simulink model "ChemicalProcessOptimization"  (R2019b)
settings: Solver=FixedStepAuto  StartTime=0  StopTime=45  FixedStep=Ts  RelTol=1e-3  EnableMultiTasking=on
PreLoadFcn:
  | Ts = 0.5;
  | load CSTRData
values from neighbouring files (symbols this model uses):
  a_vec = [0.384207621232031;0.492686723524811;0.580956543031792;0.649017079752974;0.696868333688357;0.72451030483794;0.731942993201725;0.71916639877971;0.686180521571896;0.632985361578283;0.55958091879887;0.465967193233659;0.352144184882648;0.218111893745838;0.0638703198232284]    [run_benchmark.m]
  b_vec = [0.0628087670628903;0.0875474545057933;0.110088960048547;0.130433283691153;0.148580425433609;0.164530385275917;0.178283163218075;0.189838759260085;0.199197173401946;0.206358405643658;0.211322455985221;0.214089324426636;0.214659010967901;0.213031515609018;0.209206838349985]    [run_benchmark.m]
  change_per_step_Tc_control = 2    [init_vars.m]
  conc_noise = (CrEQ(1)-CrEQ(5))*noise_magnitude    [init_vars.m]
  Cr_sim_ini = 8.57    [init_vars.m]    (also in run_benchmark.m)
  Cr_vec = [2 2.5 3 3.5 4 4.5 5 5.5 6 6.5 7 7.5 8 8.5 9]    [run_benchmark.m]
  j_scenario = 1    [init_vars.m]
  Ki_vec = [-7.98512854300473;-6.23612330817463;-4.75246287755465;-3.53414725114479;-2.58117642894504;-1.8935504109554;-1.47126919717588;-1.31433278760647;-1.42274118224718;-1.796494381098;-2.43559238415893;-3.34003519142998;-4.50982280291114;-5.94495521860242;-7.64543243850381]    [run_benchmark.m]
  Kp_vec = [-2.00046148741648;-2.3184560846763;-2.65393524901532;-3.00689898043353;-3.37734727893094;-3.76528014450754;-4.17069757716334;-4.59359957689834;-5.03398614371254;-5.49185727760593;-5.96721297857851;-6.4600532466303;-6.97037808176128;-7.49818748397146;-8.04348145326083]    [run_benchmark.m]
  Kt_vec = [3.60620000481947;3.57285570622906;3.55992955218359;3.56742154268306;3.59533167772747;3.64365995731683;3.71240638145112;3.80157095013036;3.91115366335453;4.04115452112365;4.19157352343771;4.36241067029671;4.55366596170065;4.76533939764953;4.99743097814336]    [run_benchmark.m]
  Tc_sim_ini = 297.9798    [init_vars.m]
  temp_noise = (TrEQ(1)-TrEQ(5))*noise_magnitude    [init_vars.m]
  Tr_sim_ini = 311.2612    [init_vars.m]    (also in run_benchmark.m)
undefined symbols (not defined in the file or in its folder): CrEQ, DiscIntNeverNeededParam, sigbuilder_block, TrEQ
libraries: simulink x1, bonsai_library x1
settings Model: Creator=The MathWorks, Inc.  LastModifiedBy=jomcdowe
settings DataIOCC: InitialState=[311.267; 8.5695]  LimitDataPoints=on  SaveFormat=Array  ReturnWorkspaceOutputs=off  SignalLoggingName=logsOut
settings OptimizationCC: BooleanDataType=off  DefaultParameterBehavior=Inlined  InlineInvariantSignals=on  BufferReuse=off  ExpressionDepthLimit=2147483647  InitFltsAndDblsToZero=on  LifeSpan=inf
settings DebuggingCC: SaveWithParameterizedLinksMsg=none  UnderspecifiedInitializationDetection=Classic  MergeDetectMultiDrivingBlocksExec=none  CheckExecutionContextPreStartOutputMsg=on  CheckExecutionContextRuntimeOutputMsg=on  SignalResolutionControl=TryResolveAllWithWarning  MultiTaskDSMMsg=warning  MultiTaskCondExecSysMsg=none  AllowSymbolicDim=off  StateNameClashWarn=warning  SFUnexpectedBacktrackingDiag=warning  SFNoUnconditionalDefaultTransitionDiag=warning  SFExecutionAtInitializationDiag=none  ArithmeticOperatorsInVariantConditions=warning
settings HardwareCC: ProdBitPerPointer=32  ProdBitPerSizeT=32  ProdBitPerPtrDiffT=32  ProdLargestAtomicFloat=None  ProdIntDivRoundTo=Undefined  ProdEndianess=Unspecified  ProdWordSize=32  ProdHWDeviceType=32-bit Generic  TargetUnknown=on
settings ModelReferenceCC: PropagateSignalLabelsOutOfModel=off
settings SFSimCC: SimUseLocalCustomCode=off  CustomCodeUndefinedFunction=UseInterfaceOnly
settings RTWCC: RTWUseLocalCustomCode=off
settings CodeAppCC: StateflowObjectComments=on
settings GRTTargetCC: TargetFcnLib=ansi_tfl_tmw.mat  TargetLangStandard=C89/C90 (ANSI)  CombineOutputUpdateFcns=off  GRTInterface=on
settings ConfigComp: CovMetricSettings=dw  CovSaveCumulativeToWorkspaceVar=on  CovSaveSingleToWorkspaceVar=on  CovExternalEMLEnable=off  CovSFcnEnable=off

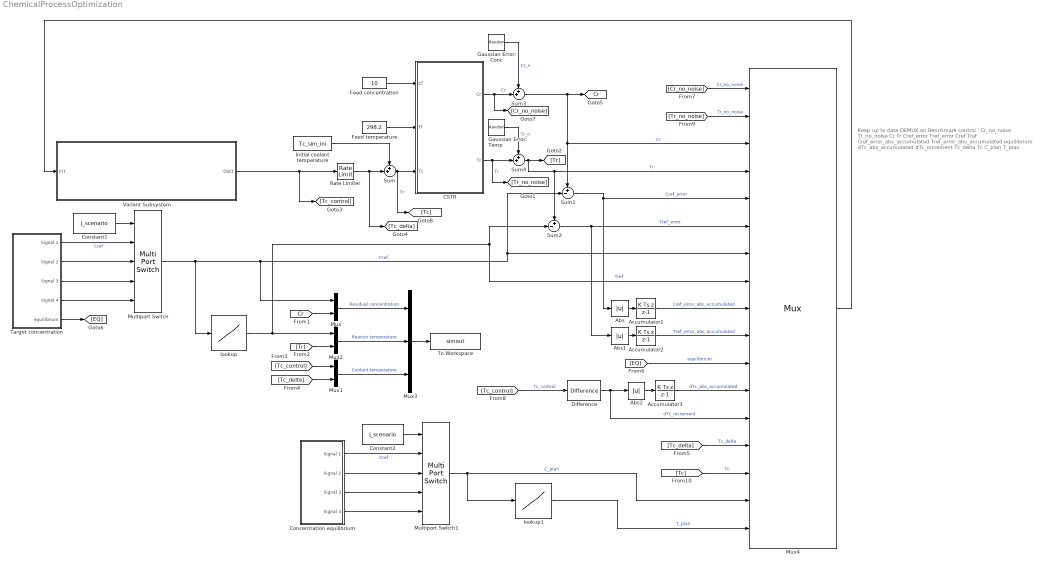
== system ChemicalProcessOptimization ==
  note: Keep up to date DEMUX on Benchmark control :
      |
      | Cr_no_noise
      | Tr_no_noise
      | Cr
      | Tr
      | Cref_error
      | Tref_error
      | Cref
      | Tref
      | Cref_error_abs_accumulated
      | Tref_error_abs_accumulated
      | equilibrium
      | dTc_abs_accumulated
      | dTc_increment
      | Tc_delta
      | Tc
      | C_plan
      | T_plan
  Abs : Abs
  Abs1 : Abs
  Abs2 : Abs
  Accumulator1 : DiscreteIntegrator  IntegratorMethod=Integration: Backward Euler  gainval=1/Ts  SampleTime=-1  ICPrevOutput=DiscIntNeverNeededParam  ICPrevScaledInput=DiscIntNeverNeededParam
  Accumulator2 : DiscreteIntegrator  IntegratorMethod=Integration: Backward Euler  gainval=1/Ts  SampleTime=-1  ICPrevOutput=DiscIntNeverNeededParam  ICPrevScaledInput=DiscIntNeverNeededParam
  Accumulator3 : DiscreteIntegrator  IntegratorMethod=Integration: Backward Euler  gainval=1/Ts  SampleTime=-1  ICPrevOutput=DiscIntNeverNeededParam  ICPrevScaledInput=DiscIntNeverNeededParam
  CSTR : Subsystem
  Concentration equilibrium : Subsystem  Tag=STV Subsys  LoadFcn=sigbuilder_block('load');  StartFcn=sigbuilder_block('start');  StopFcn=sigbuilder_block('stop');  ClipboardFcn=sigbuilder_block('clipboard');  mask(Sigbuilder block){tuvar=[0:10]}
      mask help: Simulink:masks:SigbuilderBlock_MD
      mask init:
      | if ~strcmp(get_param(bdroot(gcbh),'SimulationStatus'),'stopped') tuvar = sigbuilder_block('maskInit'); end
      settings: CopyFcn=sigbuilder_block('copy');  DeleteFcn=sigbuilder_block('delete');  ModelCloseFcn=sigbuilder_block('modelClose');  PreSaveFcn=sigbuilder_block('preSave');  PauseFcn=sigbuilder_block('pause');  ContinueFcn=sigbuilder_block('continue');  NameChangeFcn=sigbuilder_block('namechange');  OpenFcn=sigbuilder_block('open',[490.5 190.125 550.5 359.625 ]);  CloseFcn=sigbuilder_block('close');
      mask Display: plot(0, 0, 100, 100,[2, 2, 32, 32, 2], [68, 8, 8, 68, 68],[32, 2], [38, 38], [32, 19, 2],[53, 60, 44], [32, 17, 17, 2],[16, 16, 31, 31]);txt = getActiveGroup(gcbh);text(2, 100, txt,'verticalAlignment', 'top');
  Constant1 : Constant  Value=j_scenario
  Constant2 : Constant  Value=j_scenario
  Difference : simulink/Discrete/Difference  ICPrevInput=0.0  OutMin=[]  OutMax=[]  OutDataType=fixdt(1, 16)  OutScaling=2^-10  DoSatur=off
  Feed concentration : Constant  Value=10  SampleTime=0
  Feed temperature : Constant  Value=298.2  SampleTime=0
  Gaussian Error: Conc : RandomNumber  Variance=conc_noise*conc_noise  SampleTime=Ts
  Gaussian Error: Temp : RandomNumber  Variance=temp_noise*temp_noise  Seed=10  SampleTime=Ts
  Initial coolant temperature : Constant  Value=Tc_sim_ini  SampleTime=0
  Multiport Switch : MultiPortSwitch  Inputs=4
  Multiport Switch1 : MultiPortSwitch  Inputs=4
  Mux : Mux  Inputs=2
  Mux1 : Mux  Inputs=2
  Mux2 : Mux  Inputs=2
  Mux3 : Mux  Inputs=3
  Mux4 : Mux  Inputs=17
      settings: DisplayOption=signals
  Rate Limiter : RateLimiter  RisingSlewLimit=10  FallingSlewLimit=-10  SampleTimeMode=inherited
  Sum : Sum  Inputs=++|
  Sum1 : Sum  Inputs=+-|
  Sum2 : Sum  Inputs=+-|
  Sum3 : Sum  Inputs=++|
  Sum4 : Sum  Inputs=++|
  Target concentration : Subsystem  Tag=STV Subsys  LoadFcn=sigbuilder_block('load');  StartFcn=sigbuilder_block('start');  StopFcn=sigbuilder_block('stop');  ClipboardFcn=sigbuilder_block('clipboard');  mask(Sigbuilder block){tuvar=[0:10]}
      mask help: Simulink:masks:SigbuilderBlock_MD
      mask init:
      | if ~strcmp(get_param(bdroot(gcbh),'SimulationStatus'),'stopped') tuvar = sigbuilder_block('maskInit'); end
      settings: CopyFcn=sigbuilder_block('copy');  DeleteFcn=sigbuilder_block('delete');  ModelCloseFcn=sigbuilder_block('modelClose');  PreSaveFcn=sigbuilder_block('preSave');  PauseFcn=sigbuilder_block('pause');  ContinueFcn=sigbuilder_block('continue');  NameChangeFcn=sigbuilder_block('namechange');  OpenFcn=sigbuilder_block('open',[414.375 193.875 550.5 359.625 ]);  CloseFcn=sigbuilder_block('close');
      mask Display: plot(0, 0, 100, 100,[2, 2, 32, 32, 2], [68, 8, 8, 68, 68],[32, 2], [38, 38], [32, 19, 2],[53, 60, 44], [32, 17, 17, 2],[16, 16, 31, 31]);txt = getActiveGroup(gcbh);text(2, 100, txt,'verticalAlignment', 'top');
  To Workspace : ToWorkspace  VariableName=simout  SampleTime=-1
  Variant Subsystem : Subsystem  VariantControlMode=Label  Variant=on  LabelModeActiveChoice=Bonsai
  lookup : Lookup_n-D  NumberOfTableDimensions=1  LookupTableObject=''  BreakpointsForDimension1=flipud(CrEQ)  Table=flipud(TrEQ)  RndMeth=Simplest  InputSameDT=on
  lookup1 : Lookup_n-D  NumberOfTableDimensions=1  LookupTableObject=''  BreakpointsForDimension1=flipud(CrEQ)  Table=flipud(TrEQ)  RndMeth=Simplest  InputSameDT=on
  tag scope: Cr=global
  wires:
  Feed concentration/1 -> CSTR/1(Cf)
  Feed temperature/1 -> CSTR/2(Tf)
  Sum4/1 -> [Tr], Sum2/1, Mux4/4  "Tr"
  Mux1/1 -> Mux3/3  "Coolant temperature"
  Initial coolant temperature/1 -> Sum/1
  Sum3/1 -> Sum1/1, Mux4/3, [Cr]  "Cr"
  [Cr] -> Mux/2
  Mux2/1 -> Mux3/2  "Reactor temperature"
  Mux/1 -> Mux3/1  "Residual concentration"
  [Tc_control] -> Mux1/1
  [Tc_delta] -> Mux1/2
  [Tr] -> Mux2/2
  lookup/1 -> Sum2/2, Mux4/8, Mux2/1  "Tref"
  Sum/1 -> [Tc], CSTR/3(Tc)  "Tc"
  Mux3/1 -> To Workspace/1
  Rate Limiter/1 -> Sum/2, [Tc_delta]
  Multiport Switch/1 -> lookup/1, Mux/1, Sum1/2, Mux4/7  "Cref"
  Sum1/1 -> Abs/1, Mux4/5  "Cref_error"
  Sum2/1 -> Abs1/1, Mux4/6  "Tref_error"
  Constant1/1 -> Multiport Switch/1
  Target concentration/1(Signal 1) -> Multiport Switch/2  "Cref"
  Target concentration/4(Signal 4) -> Multiport Switch/5
  Target concentration/2(Signal 2) -> Multiport Switch/3
  Target concentration/3(Signal 3) -> Multiport Switch/4
  Target concentration/5(equilibrium) -> [EQ]
  [EQ] -> Mux4/11  "equilibrium"
  Abs/1 -> Accumulator1/1
  Accumulator1/1 -> Mux4/9  "Cref_error_abs_accumulated"
  Abs1/1 -> Accumulator2/1
  Accumulator2/1 -> Mux4/10  "Tref_error_abs_accumulated"
  Accumulator3/1 -> Mux4/12  "dTc_abs_accumulated"
  Abs2/1 -> Accumulator3/1
  [Tc_control] -> Difference/1  "Tc_control"
  [Tc_delta] -> Mux4/14  "Tc_delta"
  Constant2/1 -> Multiport Switch1/1
  Concentration equilibrium/1(Signal 1) -> Multiport Switch1/2  "Cref"
  Concentration equilibrium/2(Signal 2) -> Multiport Switch1/3
  Concentration equilibrium/3(Signal 3) -> Multiport Switch1/4
  Concentration equilibrium/4(Signal 4) -> Multiport Switch1/5
  Multiport Switch1/1 -> Mux4/16, lookup1/1  "C_plan"
  lookup1/1 -> Mux4/17  "T_plan"
  CSTR/1(Cr) -> [Cr_no_noise], Sum3/2  "Cr"
  Gaussian Error: Conc/1 -> Sum3/1  "Cr_n"
  CSTR/2(Tr) -> [Tr_no_noise], Sum4/2  "Tr"
  Gaussian Error: Temp/1 -> Sum4/1  "Tr_n"
  Difference/1 -> Mux4/13, Abs2/1  "dTc_increment"
  Mux4/1 -> Variant Subsystem/1(In1)
  Variant Subsystem/1(Out1) -> [Tc_control], Rate Limiter/1
  [Cr_no_noise] -> Mux4/1  "Cr_no_noise"
  [Tr_no_noise] -> Mux4/2  "Tr_no_noise"
  [Tc] -> Mux4/15  "Tc"

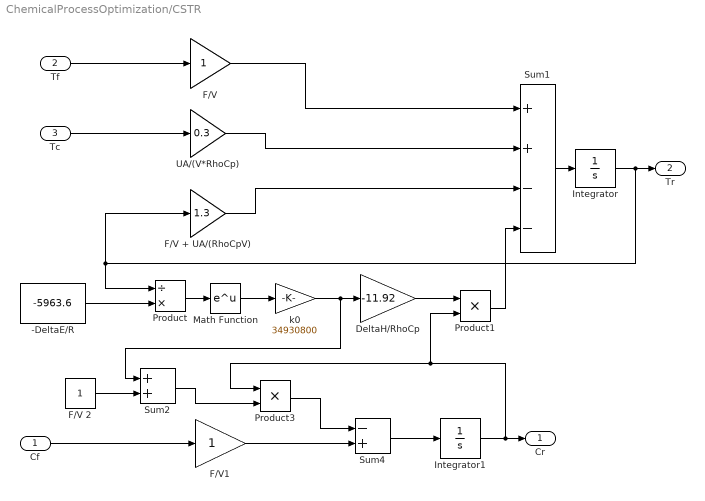
== system ChemicalProcessOptimization/CSTR ==
  Cf : Inport
  Tf : Inport  Port=2
  Tc : Inport  Port=3
  -DeltaE/R : Constant  Value=-5963.6  SampleTime=0
  DeltaH/RhoCp : Gain  Gain=-11.92  SaturateOnIntegerOverflow=on  OutDataTypeStr=Inherit: Same as input  ParamDataTypeStr=Inherit: Same as input
  F/V : Gain  SaturateOnIntegerOverflow=on  OutDataTypeStr=Inherit: Same as input  ParamDataTypeStr=Inherit: Same as input
  F/V + UA/(RhoCpV) : Gain  Gain=1.3  SaturateOnIntegerOverflow=on  OutDataTypeStr=Inherit: Same as input  ParamDataTypeStr=Inherit: Same as input
  F/V 2 : Constant  SampleTime=0
  F/V1 : Gain  SaturateOnIntegerOverflow=on  OutDataTypeStr=Inherit: Same as input  ParamDataTypeStr=Inherit: Same as input
  Integrator : Integrator  InitialCondition=Tr_sim_ini  LimitOutput=on  LowerSaturationLimit=0
  Integrator1 : Integrator  InitialCondition=Cr_sim_ini  LimitOutput=on  LowerSaturationLimit=0
  Math Function : Math  SaturateOnIntegerOverflow=on
  Product : Product  Inputs=/*  SaturateOnIntegerOverflow=on  RndMeth=Zero  InputSameDT=on  OutDataTypeStr=Inherit: Same as first input
  Product1 : Product  SaturateOnIntegerOverflow=on  RndMeth=Zero  InputSameDT=on  OutDataTypeStr=Inherit: Same as first input
  Product3 : Product  SaturateOnIntegerOverflow=on  RndMeth=Zero  InputSameDT=on  OutDataTypeStr=Inherit: Same as first input
  Sum1 : Sum  Inputs=++--  SaturateOnIntegerOverflow=on  InputSameDT=on  OutDataTypeStr=Inherit: Same as first input
  Sum2 : Sum  SaturateOnIntegerOverflow=on  InputSameDT=on  OutDataTypeStr=Inherit: Same as first input
  Sum4 : Sum  Inputs=-+  SaturateOnIntegerOverflow=on  InputSameDT=on  OutDataTypeStr=Inherit: Same as first input
  UA/(V*RhoCp) : Gain  Gain=0.3  SaturateOnIntegerOverflow=on  OutDataTypeStr=Inherit: Same as input  ParamDataTypeStr=Inherit: Same as input
  k0 : Gain  Gain=34930800  SaturateOnIntegerOverflow=on  OutDataTypeStr=Inherit: Same as input  ParamDataTypeStr=Inherit: Same as input
  Cr : Outport
  Tr : Outport  Port=2
  wires:
  F/V/1 -> Sum1/1
  Sum1/1 -> Integrator/1
  Integrator/1 -> Product/1, F/V + UA/(RhoCpV)/1, Tr/1
  UA/(V*RhoCp)/1 -> Sum1/2
  F/V + UA/(RhoCpV)/1 -> Sum1/3
  Product/1 -> Math Function/1
  Math Function/1 -> k0/1
  DeltaH/RhoCp/1 -> Product1/1
  Product1/1 -> Sum1/4
  k0/1 -> DeltaH/RhoCp/1, Sum2/1
  -DeltaE/R/1 -> Product/2
  Product3/1 -> Sum4/1
  Sum4/1 -> Integrator1/1
  Integrator1/1 -> Product1/2, Product3/1, Cr/1
  F/V 2/1 -> Sum2/2
  F/V1/1 -> Sum4/2
  Tf/1 -> F/V/1
  Cf/1 -> F/V1/1
  Tc/1 -> UA/(V*RhoCp)/1
  Sum2/1 -> Product3/2

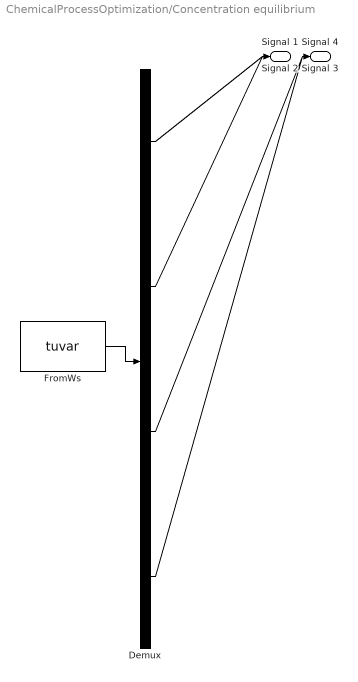
== system ChemicalProcessOptimization/Concentration equilibrium ==
  Demux : Demux  Tag=STV Demux
  FromWs : FromWorkspace  Tag=STV FromWs  VariableName=tuvar  SampleTime=0
      SigBuilderData=|
      | common.afterFinalStr = 'Extrapolate'
      | common.sampleTime = 0
      | dataSet.timeRange = [0 90]
      | dataSet.name = 'Group 1'
      | sbobj.Groups.Name = 'Group 1'
      | sbobj.Groups.Signals(1).Name = 'Signal 1'
      | sbobj.Groups.Signals(1).XData = [0 2 2 90]
      | sbobj.Groups.Signals(1).YData = [8.57 8.57 2 2]
      | sbobj.Groups.Signals(2).Name = 'Signal 2'
      | sbobj.Groups.Signals(2).XData = [0 2 2 90]
      | sbobj.Groups.Signals(2).YData = [8.57 8.57 3.6425 3.6425]
      | sbobj.Groups.Signals(3).Name = 'Signal 3'
      | sbobj.Groups.Signals(3).XData = [0 2 2 90]
      | sbobj.Groups.Signals(3).YData = [8.57 8.57 5.285 5.285]
      | sbobj.Groups.Signals(4).Name = 'Signal 4'
      | sbobj.Groups.Signals(4).XData = [0 2 2 90]
      | sbobj.Groups.Signals(4).YData = [8.57 8.57 6.9275 6.9275]
      | sbobj.Groups.TimeRange = [0 90]
  Signal 1 : Outport  Tag=STV Outport
  Signal 2 : Outport  Tag=STV Outport  Port=2
  Signal 3 : Outport  Tag=STV Outport  Port=3
  Signal 4 : Outport  Tag=STV Outport  Port=4
  wires:
  FromWs/1 -> Demux/1
  Demux/1 -> Signal 1/1
  Demux/2 -> Signal 2/1
  Demux/3 -> Signal 3/1
  Demux/4 -> Signal 4/1

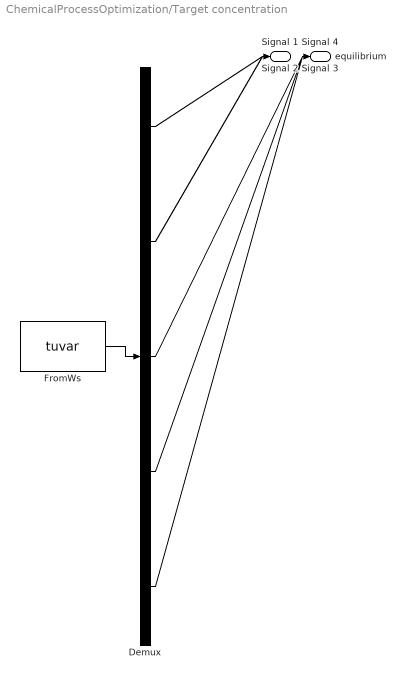
== system ChemicalProcessOptimization/Target concentration ==
  Demux : Demux  Tag=STV Demux  Outputs=5
  FromWs : FromWorkspace  Tag=STV FromWs  VariableName=tuvar  SampleTime=0
      SigBuilderData=|
      | common.afterFinalStr = 'Extrapolate'
      | common.sampleTime = 0
      | dataSet.timeRange = [0 90]
      | dataSet.name = 'Group 1'
      | sbobj.Groups.Name = 'Group 1'
      | sbobj.Groups.Signals(1).Name = 'Signal 1'
      | sbobj.Groups.Signals(1).XData = [0 2 28 90]
      | sbobj.Groups.Signals(1).YData = [8.57 8.57 2 2]
      | sbobj.Groups.Signals(2).Name = 'Signal 2'
      | sbobj.Groups.Signals(2).XData = [0 2 28 90]
      | sbobj.Groups.Signals(2).YData = [8.57 8.57 3.6425 3.6425]
      | sbobj.Groups.Signals(3).Name = 'Signal 3'
      | sbobj.Groups.Signals(3).XData = [0 2 28 90]
      | sbobj.Groups.Signals(3).YData = [8.57 8.57 5.285 5.285]
      | sbobj.Groups.Signals(4).Name = 'Signal 4'
      | sbobj.Groups.Signals(4).XData = [0 2 28 90]
      | sbobj.Groups.Signals(4).YData = [8.57 8.57 6.9275 6.9275]
      | sbobj.Groups.Signals(5).Name = 'equilibrium'
      | sbobj.Groups.Signals(5).XData = [0 2 2 28 28 90]
      | sbobj.Groups.Signals(5).YData = [1 1 0 0 1 1]
      | sbobj.Groups.TimeRange = [0 90]
  Signal 1 : Outport  Tag=STV Outport
  Signal 2 : Outport  Tag=STV Outport  Port=2
  Signal 3 : Outport  Tag=STV Outport  Port=3
  Signal 4 : Outport  Tag=STV Outport  Port=4
  equilibrium : Outport  Tag=STV Outport  Port=5
  wires:
  FromWs/1 -> Demux/1
  Demux/1 -> Signal 1/1
  Demux/2 -> Signal 2/1
  Demux/3 -> Signal 3/1
  Demux/4 -> Signal 4/1
  Demux/5 -> equilibrium/1

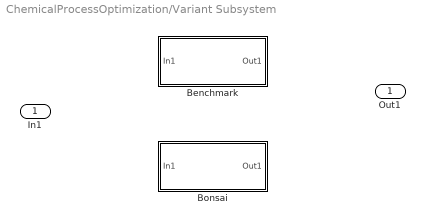
== system ChemicalProcessOptimization/Variant Subsystem ==
  In1 : Inport
  Benchmark : Subsystem  VariantControl=Benchmark
  Bonsai : Subsystem  VariantControl=Bonsai
  Out1 : Outport

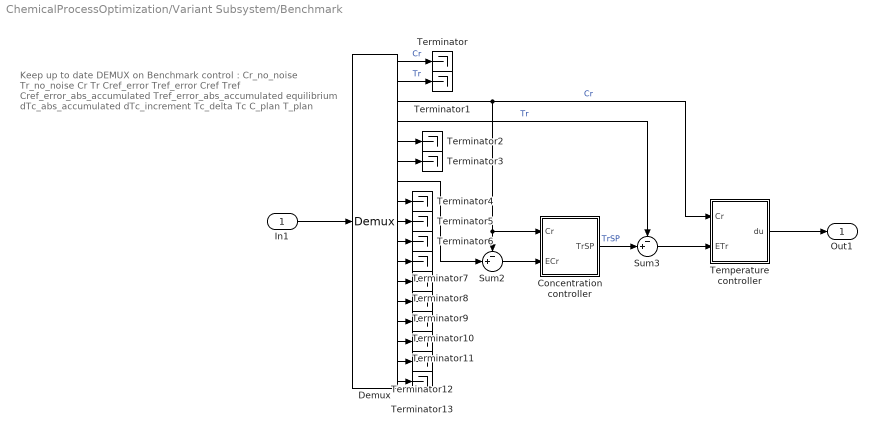
== system ChemicalProcessOptimization/Variant Subsystem/Benchmark ==
  note: Keep up to date DEMUX on Benchmark control :
      |
      | Cr_no_noise
      | Tr_no_noise
      | Cr
      | Tr
      | Cref_error
      | Tref_error
      | Cref
      | Tref
      | Cref_error_abs_accumulated
      | Tref_error_abs_accumulated
      | equilibrium
      | dTc_abs_accumulated
      | dTc_increment
      | Tc_delta
      | Tc
      | C_plan
      | T_plan
  In1 : Inport
  Concentration controller : Subsystem
  Demux : Demux  Outputs=17
  Sum2 : Sum  Inputs=-+|
  Sum3 : Sum  Inputs=-+|
  Temperature controller : Subsystem
  Terminator{,1..13} (14 alike) : Terminator
  Out1 : Outport
  wires:
  In1/1 -> Demux/1
  Sum2/1 -> Concentration controller/2(ECr)
  Concentration controller/1(TrSP) -> Sum3/2  "TrSP"
  Demux/3 -> Concentration controller/1(Cr), Sum2/1, Temperature controller/1(Cr)  "Cr"
  Sum3/1 -> Temperature controller/2(ETr)
  Demux/4 -> Sum3/1  "Tr"
  Temperature controller/1(du) -> Out1/1
  Demux/7 -> Sum2/2
  Demux/1 -> Terminator/1  "Cr"
  Demux/2 -> Terminator1/1  "Tr"
  Demux/5 -> Terminator2/1
  Demux/6 -> Terminator3/1
  Demux/8 -> Terminator4/1
  Demux/9 -> Terminator5/1
  Demux/10 -> Terminator6/1
  Demux/11 -> Terminator7/1
  Demux/12 -> Terminator8/1
  Demux/13 -> Terminator9/1
  Demux/14 -> Terminator10/1
  Demux/15 -> Terminator11/1
  Demux/16 -> Terminator12/1
  Demux/17 -> Terminator13/1

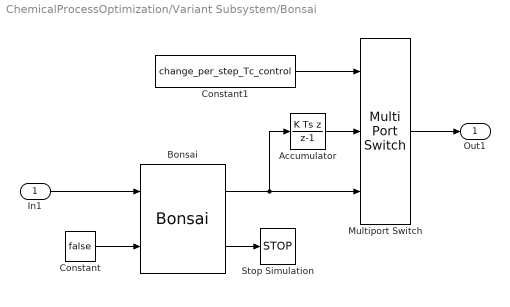
== system ChemicalProcessOptimization/Variant Subsystem/Bonsai ==
  In1 : Inport
  Accumulator : DiscreteIntegrator  IntegratorMethod=Integration: Backward Euler  gainval=1/Ts  SampleTime=-1  ICPrevOutput=DiscIntNeverNeededParam  ICPrevScaledInput=DiscIntNeverNeededParam
  Bonsai : bonsai_library/Bonsai  sampleTime=[Ts, 0]
      settings: SourceProductName=Bonsai Toolbox
  Constant : Constant  Value=false
  Constant1 : Constant  Value=change_per_step_Tc_control
  Multiport Switch : MultiPortSwitch  Inputs=2
  Stop Simulation : Stop
  Out1 : Outport
  wires:
  Constant/1 -> Bonsai/2
  Bonsai/2 -> Stop Simulation/1
  Multiport Switch/1 -> Out1/1
  In1/1 -> Bonsai/1
  Constant1/1 -> Multiport Switch/1
  Bonsai/1 -> Accumulator/1, Multiport Switch/3
  Accumulator/1 -> Multiport Switch/2

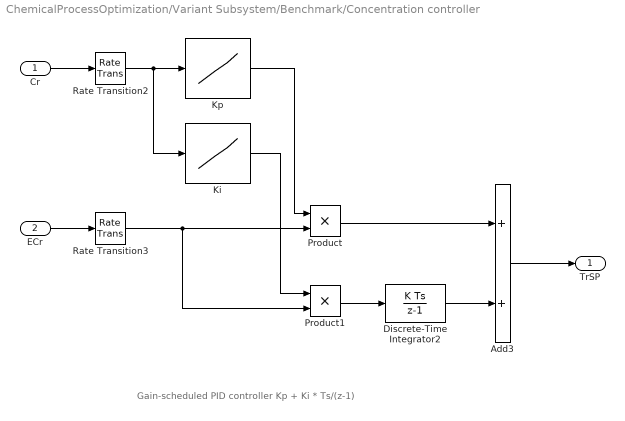
== system ChemicalProcessOptimization/Variant Subsystem/Benchmark/Concentration controller ==
  note: Gain-scheduled PID controller Kp + Ki * Ts/(z-1)
  Cr : Inport
  ECr : Inport  Port=2
  Add3 : Sum
  Discrete-Time Integrator2 : DiscreteIntegrator  InitialCondition=Tr_sim_ini  SampleTime=Ts  ICPrevOutput=DiscIntNeverNeededParam  ICPrevScaledInput=DiscIntNeverNeededParam
  Ki : Lookup_n-D  NumberOfTableDimensions=1  LookupTableObject=''  BreakpointsForDimension1=Cr_vec  Table=Ki_vec  InternalRulePriority=Speed  RndMeth=Simplest  InputSameDT=on
  Kp : Lookup_n-D  NumberOfTableDimensions=1  LookupTableObject=''  BreakpointsForDimension1=Cr_vec  Table=Kp_vec  InternalRulePriority=Speed  RndMeth=Simplest  InputSameDT=on
  Product : Product
  Product1 : Product
  Rate Transition2 : RateTransition  OutPortSampleTime=Ts
  Rate Transition3 : RateTransition  OutPortSampleTime=Ts
  TrSP : Outport
  wires:
  ECr/1 -> Rate Transition3/1
  Discrete-Time Integrator2/1 -> Add3/2
  Product/1 -> Add3/1
  Add3/1 -> TrSP/1
  Cr/1 -> Rate Transition2/1
  Kp/1 -> Product/1
  Rate Transition2/1 -> Ki/1, Kp/1
  Product1/1 -> Discrete-Time Integrator2/1
  Rate Transition3/1 -> Product1/2, Product/2
  Ki/1 -> Product1/1

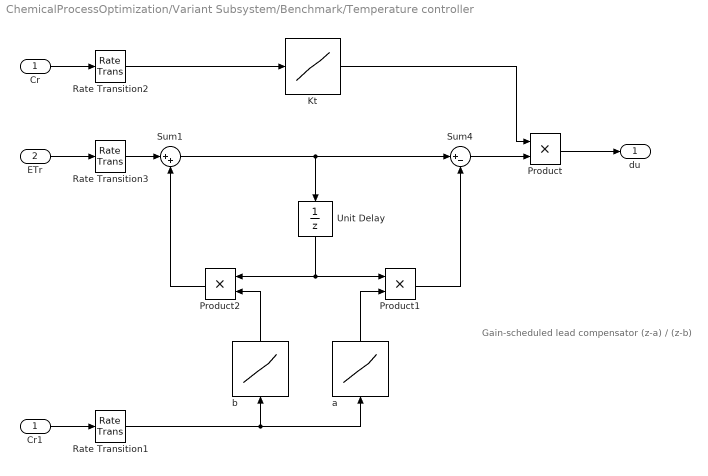
== system ChemicalProcessOptimization/Variant Subsystem/Benchmark/Temperature controller ==
  note: Gain-scheduled lead compensator
      | (z-a) / (z-b)
  Cr : Inport
  ETr : Inport  Port=2
  Cr1 : InportShadow
  Kt : Lookup_n-D  NumberOfTableDimensions=1  LookupTableObject=''  BreakpointsForDimension1=Cr_vec  Table=Kt_vec  InternalRulePriority=Speed  RndMeth=Simplest  InputSameDT=on
  Product : Product
  Product1 : Product
  Product2 : Product
  Rate Transition1 : RateTransition  OutPortSampleTime=Ts
  Rate Transition2 : RateTransition  OutPortSampleTime=Ts
  Rate Transition3 : RateTransition  OutPortSampleTime=Ts
  Sum1 : Sum  Inputs=|++
  Sum4 : Sum  Inputs=|+-
  Unit Delay : UnitDelay  SampleTime=Ts  HasFrameUpgradeWarning=on
  a : Lookup_n-D  NumberOfTableDimensions=1  LookupTableObject=''  BreakpointsForDimension1=Cr_vec  Table=a_vec  InternalRulePriority=Speed  RndMeth=Simplest  InputSameDT=on
  b : Lookup_n-D  NumberOfTableDimensions=1  LookupTableObject=''  BreakpointsForDimension1=Cr_vec  Table=b_vec  InternalRulePriority=Speed  RndMeth=Simplest  InputSameDT=on
  du : Outport
  wires:
  Product/1 -> du/1
  Product1/1 -> Sum4/2
  Sum1/1 -> Sum4/1, Unit Delay/1
  Sum4/1 -> Product/2
  Product2/1 -> Sum1/2
  Unit Delay/1 -> Product1/1, Product2/1
  ETr/1 -> Rate Transition3/1
  Rate Transition3/1 -> Sum1/1
  Cr/1 -> Rate Transition2/1
  Rate Transition2/1 -> Kt/1
  Kt/1 -> Product/1
  Cr1/1 -> Rate Transition1/1
  a/1 -> Product1/2
  Rate Transition1/1 -> b/1, a/1
  b/1 -> Product2/2
